simulink model "basic_pid_fixed_spring"  (R2015a)
settings: Solver=ode45  StartTime=0.0  StopTime=10.0  RelTol=1e-3
undefined symbols (not defined in the file): b_L, b_m, g, J_L, J_m, k_1, k_2, K_a, K_d, K_i, K_p, K_t, l, m, N, pid, theta_c
libraries: simulink x2
settings Model: Creator=preston  LastModifiedBy=preston

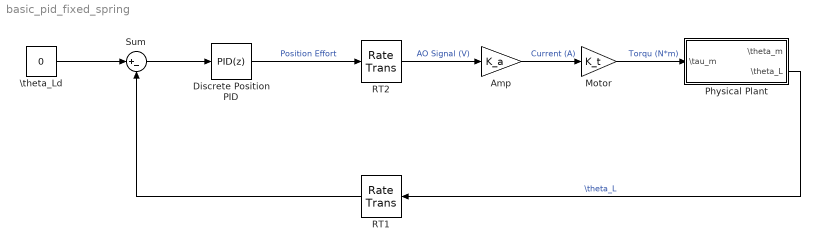
== system basic_pid_fixed_spring ==
  Amp : Gain  Gain=K_a
  Discrete Position PID : simulink/Continuous/PID Controller  Controller=PID  TimeDomain=Discrete-time  SampleTime=-1  IntegratorMethod=Backward Euler  FilterMethod=Forward Euler  Form=Parallel  UseFilter=off  ControllerParametersSource=internal  P=K_p  I=K_i  D=K_d  N=pid.N  InitialConditionSource=internal  InitialConditionForIntegrator=0  InitialConditionForFilter=0  ExternalReset=none  LimitOutput=off  UpperSaturationLimit=inf  LowerSaturationLimit=-inf  LinearizeAsGain=off  AntiWindupMode=none  Kb=1  TrackingMode=off  Kt=1  PParamMin=[]  PParamMax=[]  IParamMin=[]  IParamMax=[]  DParamMin=[]  DParamMax=[]  NParamMin=[]  NParamMax=[]  KbParamMin=[]  KbParamMax=[]  KtParamMin=[]  KtParamMax=[]  POutMin=[]  POutMax=[]  IOutMin=[]  IOutMax=[]  DOutMin=[]  DOutMax=[]  NOutMin=[]  NOutMax=[]  KbOutMin=[]  KbOutMax=[]  KtOutMin=[]  KtOutMax=[]  IntegratorOutMin=[]  IntegratorOutMax=[]  FilterOutMin=[]  FilterOutMax=[]  SumOutMin=[]  SumOutMax=[]  SumI1OutMin=[]  SumI1OutMax=[]  SumI2OutMin=[]  SumI2OutMax=[]  SumI3OutMin=[]  SumI3OutMax=[]  SumDOutMin=[]  SumDOutMax=[]  SaturationOutMin=[]  SaturationOutMax=[]  IntegratorContinuousStateAttributes=''  IntegratorStateMustResolveToSignalObject=off  IntegratorRTWStateStorageClass=Auto  FilterContinuousStateAttributes=''  FilterStateMustResolveToSignalObject=off  FilterRTWStateStorageClass=Auto  DifferentiatorICPrevScaledInput=0  DifferentiatorOutMin=[]  DifferentiatorOutMax=[]
  Motor : Gain  Gain=K_t
  "Physical Plant " : Subsystem
  RT1 : RateTransition  OutPortSampleTime=T_sample_control
  RT2 : RateTransition
  Sum : Sum  Inputs=|+-
  \theta_Ld : Constant  Value=0
  wires:
  "Physical Plant "/2(\theta_L) -> RT1/1  "\\theta_L"
  RT2/1 -> Amp/1  "AO Signal (V)"
  Discrete Position PID/1 -> RT2/1  "Position Effort"
  \theta_Ld/1 -> Sum/1
  RT1/1 -> Sum/2
  Sum/1 -> Discrete Position PID/1
  Amp/1 -> Motor/1  "Current (A)"
  Motor/1 -> "Physical Plant "/1(\tau_m)  "Torqu (N*m)"

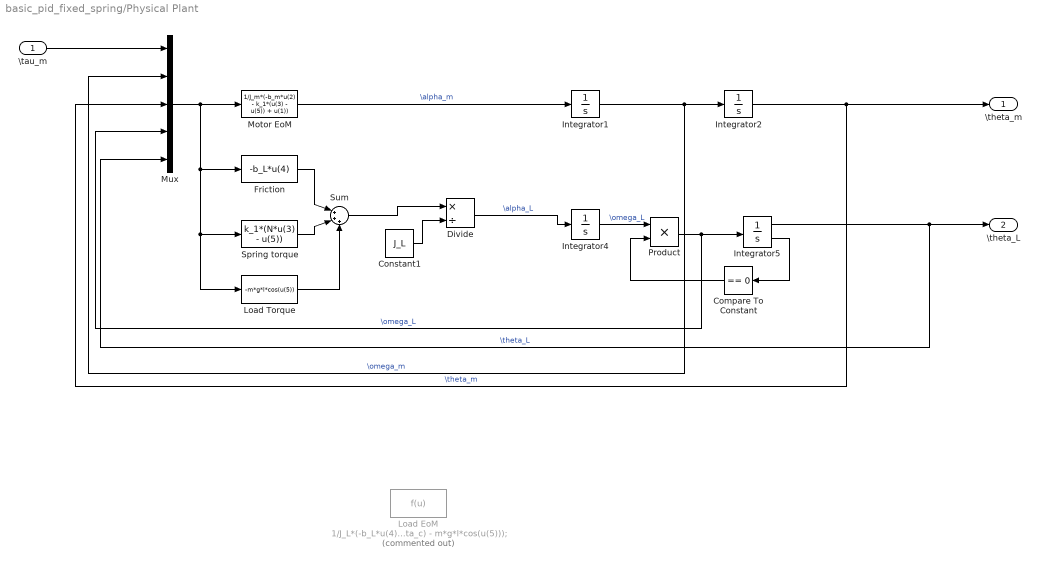
== system basic_pid_fixed_spring/Physical Plant  ==
  \tau_m : Inport
  Compare To Constant : simulink/Logic and Bit Operations/Compare To Constant  relop===  const=0  OutDataTypeStr=boolean
  Constant1 : Constant  Value=J_L
  Divide : Product  Inputs=*/
  Friction : Fcn  Expr=-b_L*u(4)
  Integrator1 : Integrator
  Integrator2 : Integrator
  Integrator4 : Integrator
  Integrator5 : Integrator  LimitOutput=on  UpperSaturationLimit=pi/4  LowerSaturationLimit=-pi/4  ShowSaturationPort=on
  Load EoM : Fcn  Commented=on  Expr=1/J_L*(-b_L*u(4) + k_1*(u(3) - u(5)) - k_2*(u(5) - theta_c) - m*g*l*cos(u(5)));
  Load Torque : Fcn  Expr=-m*g*l*cos(u(5))
  Motor EoM : Fcn  Expr=1/J_m*(-b_m*u(2) - k_1*(u(3) - u(5)) + u(1))
  Mux : Mux  Inputs=5
  Product : Product
  Spring torque : Fcn  Expr=k_1*(N*u(3) - u(5))
  Sum : Sum  Inputs=|+++
  "\\theta_m " : Outport
  \theta_L : Outport  Port=2
  wires:
  Motor EoM/1 -> Integrator1/1  "\\alpha_m"
  Divide/1 -> Integrator4/1  "\\alpha_L"
  Integrator5/1 -> \theta_L/1, Mux/5  "\\theta_L"
  Mux/1 -> Spring torque/1, Load Torque/1, Friction/1, Motor EoM/1
  \tau_m/1 -> Mux/1
  Constant1/1 -> Divide/2
  Sum/1 -> Divide/1
  Friction/1 -> Sum/1
  Spring torque/1 -> Sum/2
  Load Torque/1 -> Sum/3
  Integrator5/2 -> Compare To Constant/1
  Integrator4/1 -> Product/1  "\\omega_L"
  Compare To Constant/1 -> Product/2
  Product/1 -> Integrator5/1, Mux/4  "\\omega_L"
  Integrator1/1 -> Mux/2, Integrator2/1  "\\omega_m"
  Integrator2/1 -> Mux/3, "\\theta_m "/1  "\\theta_m"
